simulink model "R_WR_S_block"  (R2021a)
settings: Solver=VariableStepAuto  StartTime=0.0  StopTime=10.0  RelTol=1e-3
settings Model: Creator=Nabil  LastModifiedBy=Nabil

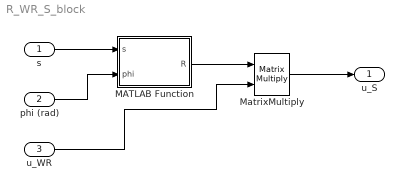
== system R_WR_S_block ==
  s : Inport
  phi (rad) : Inport  Port=2
  u_WR : Inport  Port=3  PortDimensions=3
  MATLAB Function : MATLAB Function  TreatAsAtomicUnit=on
  MatrixMultiply : Product  Multiplication=Matrix(*)
  u_S : Outport
  wires:
  u_WR/1 -> MatrixMultiply/2
  MatrixMultiply/1 -> u_S/1
  s/1 -> MATLAB Function/1(s)
  phi (rad)/1 -> MATLAB Function/2(phi)
  MATLAB Function/1(R) -> MatrixMultiply/1

== matlab function R_WR_S_block/MATLAB Function ==
  data: s input; R output; phi input
function R = fcn(s, phi)

R = R_WR_S(s, phi);
